simulink model "week1_problem3_2005052"  (R2021a)
settings: Solver=VariableStepAuto  StartTime=0.0  StopTime=0.01  RelTol=1e-3
model workspace (MAT data in the model file):
  a1 = 0.01584
  b0 = 0.5792
  b1 = -0.5792
settings Model: Creator=admin  LastModifiedBy=admin
settings SolverCC: AlgebraicLoopSolver=TrustRegion
settings DebuggingCC: SFMachineParentedDataDiag=warning

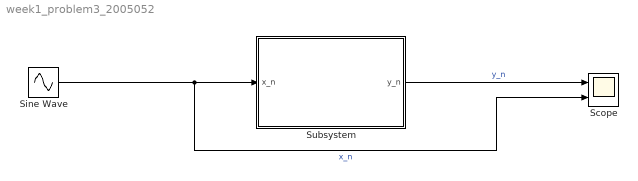
== system week1_problem3_2005052 ==
  Scope : Scope  NumInputPorts=2
  Sine Wave : Sin  Frequency=1000*pi*4  Samples=5000  SampleTime=1/5000
  Subsystem : Subsystem
  wires:
  Subsystem/1(y_n) -> Scope/1  "y_n"
  Sine Wave/1 -> Scope/2, Subsystem/1(x_n)  "x_n"

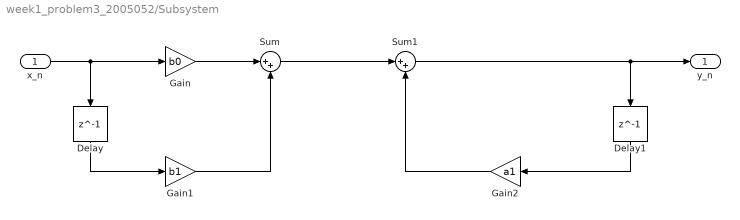
== system week1_problem3_2005052/Subsystem ==
  x_n : Inport
  Delay : Delay  DelayLength=1
  Delay1 : Delay  DelayLength=1
  Gain : Gain  Gain=b0
  Gain1 : Gain  Gain=b1
  Gain2 : Gain  Gain=a1
  Sum : Sum  Inputs=|++
  Sum1 : Sum  Inputs=|++
  y_n : Outport
  wires:
  x_n/1 -> Gain/1, Delay/1
  Delay/1 -> Gain1/1
  Gain/1 -> Sum/1
  Gain1/1 -> Sum/2
  Sum/1 -> Sum1/1
  Sum1/1 -> Delay1/1, y_n/1
  Delay1/1 -> Gain2/1
  Gain2/1 -> Sum1/2
